simulink model "No_load"  (R2022b)
settings: Solver=VariableStepAuto  StartTime=0.0  StopTime=15  RelTol=1e-3
libraries: spsDiodeLib x7, spsVoltageMeasurementLib x4, spsACVoltageSourceLib x3, spsCurrentMeasurementLib x3, simulink x2, spsMeanLib x2, spsRMSLib x2, spsDCMachineLib x1, spsDCVoltageSourceLib x1, spsIGBTLib x1, spsSeriesRLCBranchLib x1, spspowerguiLib x1
settings Model: Creator=tunaa  LastModifiedBy=tunaa

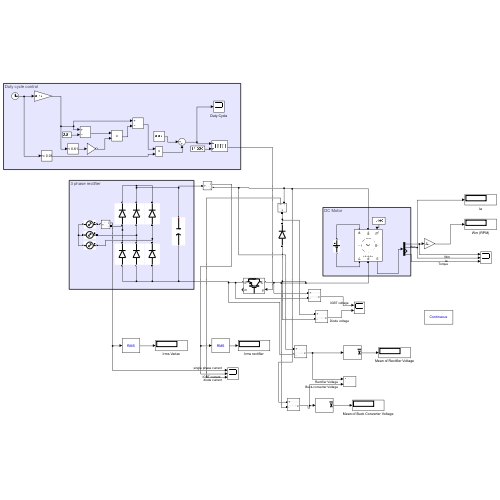
[thumbnail: Simulink's stored preview of the top-level diagram]
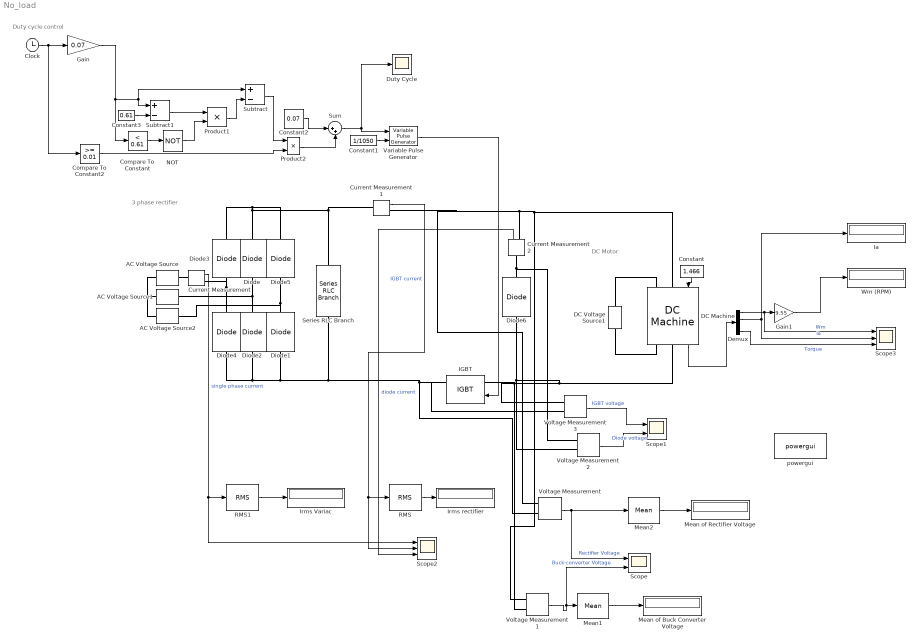
== system No_load ==
  note: DC Motor
  note: 3 phase rectifier
  note: Duty cycle control
  AC Voltage Source : spsACVoltageSourceLib/AC Voltage Source  Amplitude=136  Phase=0  Frequency=50  SampleTime=0  Measurements=None  BusType=swing  Pref=10e3  Qref=0  Qmin=-inf  Qmax=+inf
  AC Voltage Source1 : spsACVoltageSourceLib/AC Voltage Source  Amplitude=136  Phase=-120  Frequency=50  SampleTime=0  Measurements=None  BusType=swing  Pref=10e3  Qref=0  Qmin=-inf  Qmax=+inf
  AC Voltage Source2 : spsACVoltageSourceLib/AC Voltage Source  Amplitude=136  Phase=-240  Frequency=50  SampleTime=0  Measurements=None  BusType=swing  Pref=10e3  Qref=0  Qmin=-inf  Qmax=+inf
  Clock : Clock
  Compare To Constant : simulink/Logic and Bit Operations/Compare To Constant  relop=<  const=0.61  OutDataTypeStr=boolean
  Compare To Constant2 : simulink/Logic and Bit Operations/Compare To Constant  relop=>=  const=0.01  OutDataTypeStr=boolean
  Constant : Constant  Value=1.466
  Constant1 : Constant  Value=1/1050
  Constant2 : Constant  Value=0.07
  Constant3 : Constant  Value=0.61
  Current Measurement : spsCurrentMeasurementLib/Current Measurement  PhasorSimulation=off  OutputType=Complex  PSBequivalent=0
  Current Measurement1 : spsCurrentMeasurementLib/Current Measurement  PhasorSimulation=off  OutputType=Complex  PSBequivalent=0
  Current Measurement2 : spsCurrentMeasurementLib/Current Measurement  PhasorSimulation=off  OutputType=Complex  PSBequivalent=0
  DC Machine : spsDCMachineLib/DC Machine  PresetModel=No  MechanicalLoad=Torque TL  FieldType=Wound  ShowDetailedParameters=on  MeasurementBus=off  RLa="[ 0.8  0.0125]"  RLf="[ 210  23]"  Laf=1.185  MachineConstant=Torque constant (N.m/A)  Ke=1.8  Kt=1.8  J=1  Bm=0  Tf=0  w0=0  Ifinit=0.857142857142857  TsPowergui=0  TsBlock=-1
  DC Voltage Source1 : spsDCVoltageSourceLib/DC Voltage Source  Amplitude=180  Measurements=None
  Demux : Demux
  Diode{,1..6} (7 alike) : spsDiodeLib/Diode  Ron=0.001  Lon=0  Vf=0.8  IC=0  UseSnubber=0  Rs=0  Cs=0  Measurements=off
  Duty Cycle : Scope
  Gain : Gain  Gain=0.07
  Gain1 : Gain  Gain=9.55
  IGBT : spsIGBTLib/IGBT  Ron=0.001  Lon=0  Vf=1  Tf=1e-6  Tt=2e-6  IC=0  Rs=1e5  Cs=inf  Measurements=on
  Ia : Display
  Irms Variac : Display
  Irms rectifier : Display
  Mean of Buck Converter Voltage : Display
  Mean of Rectifier Voltage : Display
  Mean1 : spsMeanLib/Mean  Freq=50  Vinit=0  Ts=0
  Mean2 : spsMeanLib/Mean  Freq=50  Vinit=0  Ts=0
  NOT : Logic  Operator=NOT  IconShape=distinctive  AllPortsSameDT=off  OutDataTypeStr=boolean
  Product1 : Product
  Product2 : Product
  RMS : spsRMSLib/RMS  TrueRMS=on  Freq=50  RMSInit=0  Ts=0
  RMS1 : spsRMSLib/RMS  TrueRMS=on  Freq=50  RMSInit=0  Ts=0
  Scope : Scope  NumInputPorts=2
  Scope1 : Scope  NumInputPorts=2
  Scope2 : Scope  NumInputPorts=3
  Scope3 : Scope  NumInputPorts=3
  Series RLC Branch : spsSeriesRLCBranchLib/Series RLC Branch  LConnTagsString=__new0  RConnTagsString=__new0  BranchType=C  Resistance=1  Inductance=1e-3  SetiL0=off  InitialCurrent=0  Capacitance=470*2e-6  Setx0=off  InitialVoltage=0  Measurements=None
  Subtract : Sum  Inputs=+-
  Subtract1 : Sum  Inputs=+-
  Sum : Sum  Inputs=|++
  Variable Pulse Generator : VariablePulseGenerator  SampleTime=0.1
  Voltage Measurement{,1..3} (4 alike) : spsVoltageMeasurementLib/Voltage Measurement  PhasorSimulation=off  OutputType=Complex  PSBequivalent=0
  Wm (RPM) : Display
  powergui : spspowerguiLib/powergui  Priority=1  SimulationMode=Continuous  SampleTime=50e-6  frequency=60  Iterations=50  frequencyindice=50  Pbase=100e6  ErrMax=1e-4  UnitsV=kV  UnitsW=MW  buscounter=0  FunctionMessages=off  echomessages=off  EnableUseOfTLC=off  CurrentSourceSwitches=off  DisableSnubberDevices=off  DisableRonSwitches=off  DisableVfSwitches=off  DisplayEquations=off  AutomaticDiscreteSolvers=off  SolverType=Tustin/Backward Euler (TBE)  Interpol=off  ExternalGateDelay=off  methode=off  Ts=100  x0status=blocks  SPID=on  SwTol=0  HookPort=off  NonlinearTolerance=1e-4  nMaxIteration=100  ContinueOnMaxIteration=off  RestoreLinks=warning  ResistiveCurrentMeasurement=off  Frange=[0:2:500]  Ylog=off  Xlog=on  ShowGrid=off  save=off  variable=ZData  structure=0  ZoomFFT=off  StartTime=0.0  cycles=1  DisplayStyle=1  fundamental=60  FreqAxis=off  MaxFrequency=1000  frequencyindicesteady=1  RmsSteady=1  display=off
  wires:
  Demux/1 -> Scope3/1, Gain1/1  "Wm"
  Voltage Measurement/1 -> Scope/1, Mean2/1  "Rectifier Voltage"
  Demux/2 -> Ia/1, Scope3/2  "Ia"
  Mean2/1 -> Mean of Rectifier Voltage/1
  DC Machine/1 -> Demux/1
  Mean1/1 -> Mean of Buck Converter Voltage/1
  Voltage Measurement1/1 -> Scope/2, Mean1/1  "Buck-converter Voltage"
  Constant/1 -> DC Machine/1
  Clock/1 -> Gain/1, Compare To Constant2/1
  Constant2/1 -> Sum/1
  Constant1/1 -> Variable Pulse Generator/2
  Compare To Constant/1 -> NOT/1
  Product1/1 -> Subtract/2
  Constant3/1 -> Subtract1/2
  Subtract1/1 -> Product1/1
  NOT/1 -> Product1/2
  Gain/1 -> Compare To Constant/1, Subtract/1, Subtract1/1
  Subtract/1 -> Product2/1
  Compare To Constant2/1 -> Product2/2
  Product2/1 -> Sum/2
  Current Measurement/1 -> Scope2/1, RMS1/1  "single phase current"
  Current Measurement1/1 -> Scope2/2, RMS/1  "IGBT current"
  RMS/1 -> Irms rectifier/1
  RMS1/1 -> Irms Variac/1
  Gain1/1 -> Wm (RPM)/1
  Current Measurement2/1 -> Scope2/3  "diode current"
  Voltage Measurement2/1 -> Scope1/2  "Diode voltage"
  Voltage Measurement3/1 -> Scope1/1  "IGBT voltage"
  Demux/4 -> Scope3/3  "Torque"
  Sum/1 -> Duty Cycle/1, Variable Pulse Generator/1
  Variable Pulse Generator/1 -> IGBT/1
  connections:
  AC Voltage Source/LConn1 -- AC Voltage Source2/LConn1 -- AC Voltage Source1/LConn1
  Diode4/RConn1 -- Current Measurement/RConn1 -- Diode3/LConn1
  AC Voltage Source1/RConn1 -- Diode2/RConn1 -- Diode/LConn1
  AC Voltage Source2/RConn1 -- Diode1/RConn1 -- Diode5/LConn1
  Diode4/LConn1 -- Diode2/LConn1 -- Voltage Measurement3/LConn2 -- IGBT/RConn1 -- Voltage Measurement/LConn2 -- Series RLC Branch/RConn1 -- Diode1/LConn1
  DC Voltage Source1/RConn1 -- DC Machine/LConn2
  DC Voltage Source1/LConn1 -- DC Machine/RConn2
  Current Measurement/LConn1 -- AC Voltage Source/RConn1
  Voltage Measurement1/LConn1 -- DC Machine/LConn1 -- Current Measurement1/RConn1 -- Voltage Measurement/LConn1 -- Current Measurement2/RConn1
  Voltage Measurement2/LConn1 -- Current Measurement2/LConn1 -- Diode6/RConn1
  Series RLC Branch/LConn1 -- Current Measurement1/LConn1 -- Diode5/RConn1 -- Diode3/RConn1 -- Diode/RConn1
  Voltage Measurement2/LConn2 -- Diode6/LConn1 -- Voltage Measurement3/LConn1 -- IGBT/LConn1 -- Voltage Measurement1/LConn2 -- DC Machine/RConn1
